simulink model "logic_circuit"  (R2024b)
settings: Solver=VariableStepAuto  StartTime=0.0  StopTime=10.0  RelTol=1e-3
settings Model: Creator=chenzeyuan  LastModifiedBy=chenzeyuan

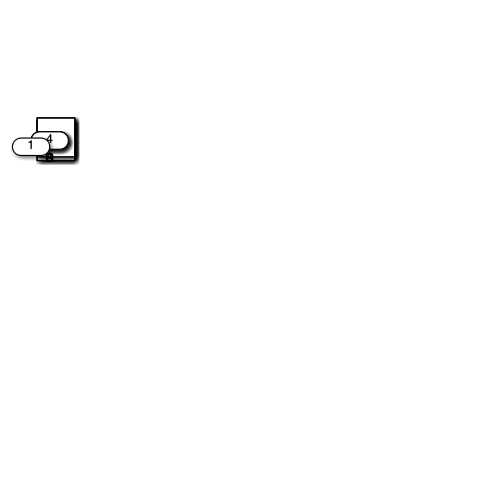
[thumbnail: Simulink's stored preview of the top-level diagram]
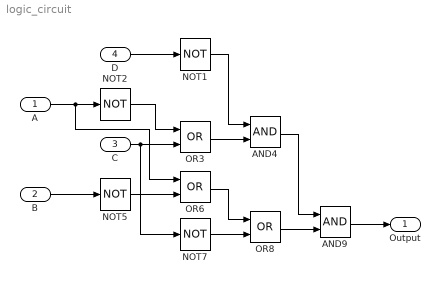
== system logic_circuit ==
  A : Inport  OutDataTypeStr=boolean
  B : Inport  Port=2  OutDataTypeStr=boolean
  C : Inport  Port=3  OutDataTypeStr=boolean
  D : Inport  Port=4  OutDataTypeStr=boolean
  AND4 : Logic  AllPortsSameDT=off  OutDataTypeStr=boolean
  AND9 : Logic  AllPortsSameDT=off  OutDataTypeStr=boolean
  NOT{1..2,5,7} (4 alike) : Logic  Operator=NOT  AllPortsSameDT=off  OutDataTypeStr=boolean
  OR3 : Logic  Operator=OR  AllPortsSameDT=off  OutDataTypeStr=boolean
  OR6 : Logic  Operator=OR  AllPortsSameDT=off  OutDataTypeStr=boolean
  OR8 : Logic  Operator=OR  AllPortsSameDT=off  OutDataTypeStr=boolean
  Output : Outport  OutDataTypeStr=boolean
  wires:
  AND9/1 -> Output/1
  OR6/1 -> OR8/1
  OR3/1 -> AND4/2
  NOT1/1 -> AND4/1
  D/1 -> NOT1/1
  NOT5/1 -> OR6/2
  NOT2/1 -> OR3/1
  OR8/1 -> AND9/2
  C/1 -> NOT7/1, OR3/2
  B/1 -> NOT5/1
  AND4/1 -> AND9/1
  NOT7/1 -> OR8/2
  A/1 -> NOT2/1, OR6/1
